simulink model "lorenz84Ver"  (R2020a)
settings: Solver=VariableStepAuto  StartTime=0.0  StopTime=25/1e5  RelTol=1e-3
undefined symbols (not defined in the file): AXI4, Lite
libraries: xbsIndex_r4 x114
settings Model: Creator=yxb20126  LastModifiedBy=yxb20126

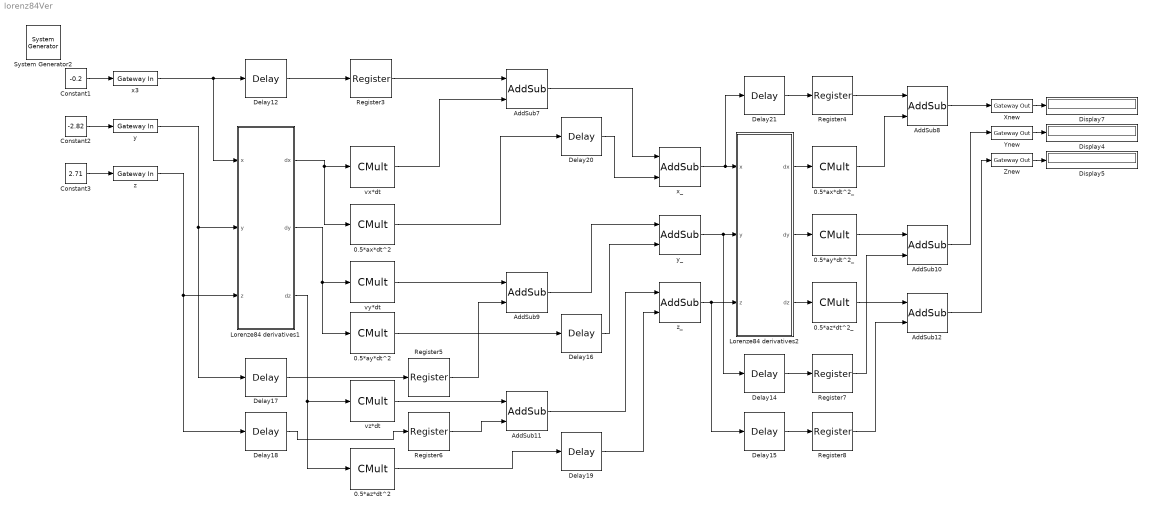
== system lorenz84Ver ==
  " System Generator2" : xbsIndex_r4/ System Generator  Tag=genX  xilinxfamily=zynq  part=xc7z020  speed=-1  package=clg400  synthesis_tool=Vivado  clock_wrapper=Clock Enables  directory=./netlist  proj_type=Vivado  Synth_file=Vivado Synthesis Defaults  Impl_file=Vivado Implementation Defaults  testbench=off  simulink_period=1/100e6  sysclk_period=10  dcm_input_clock_period=10  incr_netlist=off  trim_vbits=Everywhere in SubSystem  dbl_ovrd=According to Block Masks  core_generation=According to Block Masks  run_coregen=off  deprecated_control=off  eval_field=0  block_type=sysgen
  0.5*ax*dt^2 : xbsIndex_r4/CMult  const=5e-5  gui_display_data_type=Fixed-point  const_n_bits=32  const_bin_pt=24  float_type=Double  exp_bits=8  fraction_bits=24  en=off  latency=1  precision=User Defined  arith_type="Signed  (2's comp)"  n_bits=32  bin_pt=24  quantization=Truncate  overflow=Wrap  use_behavioral_HDL=off  mem_type=Distributed RAM  pipeline=off  dbl_ovrd=off  block_type=cmult
  0.5*ax*dt^2_ : xbsIndex_r4/CMult  const=5e-5  gui_display_data_type=Fixed-point  const_n_bits=32  const_bin_pt=24  float_type=Double  exp_bits=8  fraction_bits=24  en=off  latency=1  precision=User Defined  arith_type="Signed  (2's comp)"  n_bits=32  bin_pt=24  quantization=Truncate  overflow=Wrap  use_behavioral_HDL=off  mem_type=Distributed RAM  pipeline=off  dbl_ovrd=off  block_type=cmult
  0.5*ay*dt^2 : xbsIndex_r4/CMult  const=5e-5  gui_display_data_type=Fixed-point  const_n_bits=32  const_bin_pt=24  float_type=Double  exp_bits=8  fraction_bits=24  en=off  latency=1  precision=User Defined  arith_type="Signed  (2's comp)"  n_bits=32  bin_pt=24  quantization=Truncate  overflow=Wrap  use_behavioral_HDL=off  mem_type=Distributed RAM  pipeline=off  dbl_ovrd=off  block_type=cmult
  0.5*ay*dt^2_ : xbsIndex_r4/CMult  const=5e-5  gui_display_data_type=Fixed-point  const_n_bits=32  const_bin_pt=24  float_type=Double  exp_bits=8  fraction_bits=24  en=off  latency=1  precision=User Defined  arith_type="Signed  (2's comp)"  n_bits=32  bin_pt=24  quantization=Truncate  overflow=Wrap  use_behavioral_HDL=off  mem_type=Distributed RAM  pipeline=off  dbl_ovrd=off  block_type=cmult
  0.5*az*dt^2 : xbsIndex_r4/CMult  const=5e-5  gui_display_data_type=Fixed-point  const_n_bits=32  const_bin_pt=24  float_type=Double  exp_bits=8  fraction_bits=24  en=off  latency=1  precision=User Defined  arith_type="Signed  (2's comp)"  n_bits=32  bin_pt=24  quantization=Truncate  overflow=Wrap  use_behavioral_HDL=off  mem_type=Distributed RAM  pipeline=off  dbl_ovrd=off  block_type=cmult
  0.5*az*dt^2_ : xbsIndex_r4/CMult  const=5e-5  gui_display_data_type=Fixed-point  const_n_bits=32  const_bin_pt=24  float_type=Double  exp_bits=8  fraction_bits=24  en=off  latency=1  precision=User Defined  arith_type="Signed  (2's comp)"  n_bits=32  bin_pt=24  quantization=Truncate  overflow=Wrap  use_behavioral_HDL=off  mem_type=Distributed RAM  pipeline=off  dbl_ovrd=off  block_type=cmult
  AddSub{7..12} (6 alike) : xbsIndex_r4/AddSub  mode=Addition  use_carryin=off  use_carryout=off  en=off  latency=1  precision=User Defined  arith_type="Signed  (2's comp)"  n_bits=32  bin_pt=24  quantization=Truncate  overflow=Wrap  use_behavioral_HDL=off  hw_selection=Fabric  pipelined=off  dbl_ovrd=off  block_type=addsub
  Constant1 : Constant  Value=-0.2
  Constant2 : Constant  Value=-2.82
  Constant3 : Constant  Value=2.71
  Delay{12,14..15,17..18,21} (6 alike) : xbsIndex_r4/Delay  rst=off  infoeditControl=Selection of Reset will increase slice count due to use of real FFs and instead of SRLs  en=off  latency=15  reg_retiming=off  dbl_ovrd=off  block_type=delay
  Delay16 : xbsIndex_r4/Delay  rst=off  infoeditControl=Selection of Reset will increase slice count due to use of real FFs and instead of SRLs  en=off  latency=1  reg_retiming=off  dbl_ovrd=off  block_type=delay
  Delay19 : xbsIndex_r4/Delay  rst=off  infoeditControl=Selection of Reset will increase slice count due to use of real FFs and instead of SRLs  en=off  latency=1  reg_retiming=off  dbl_ovrd=off  block_type=delay
  Delay20 : xbsIndex_r4/Delay  rst=off  infoeditControl=Selection of Reset will increase slice count due to use of real FFs and instead of SRLs  en=off  latency=1  reg_retiming=off  dbl_ovrd=off  block_type=delay
  Display4 : Display
  Display5 : Display
  Display7 : Display
  Lorenze84 derivatives1 : Subsystem
  Lorenze84 derivatives2 : Subsystem
  Register{3..8} (6 alike) : xbsIndex_r4/Register  init=0  rst=off  en=off  dbl_ovrd=off  block_type=register
  Xnew : xbsIndex_r4/Gateway Out  inherit_from_input=off  hdl_port=on  rows=1  columns=1  UseAsDAC=off  DACChannel='1'  interface=AXI4-Lite  automatic_assignment=on  address_offset=hex2dec('00')  intf_name=''  intf_description=''  timing_constraint=None  locs_specified=off  LOCs={}  io_standard={}  block_type=gatewayout
  Ynew : xbsIndex_r4/Gateway Out  inherit_from_input=off  hdl_port=on  rows=1  columns=1  UseAsDAC=off  DACChannel='1'  interface=AXI4-Lite  automatic_assignment=on  address_offset=hex2dec('00')  intf_name=''  intf_description=''  timing_constraint=None  locs_specified=off  LOCs={}  io_standard={}  block_type=gatewayout
  Znew : xbsIndex_r4/Gateway Out  inherit_from_input=off  hdl_port=on  rows=1  columns=1  UseAsDAC=off  DACChannel='1'  interface=AXI4-Lite  automatic_assignment=on  address_offset=hex2dec('00')  intf_name=''  intf_description=''  timing_constraint=None  locs_specified=off  LOCs={}  io_standard={}  block_type=gatewayout
  vx*dt : xbsIndex_r4/CMult  const=0.01  gui_display_data_type=Fixed-point  const_n_bits=32  const_bin_pt=24  float_type=Double  exp_bits=8  fraction_bits=24  en=off  latency=1  precision=User Defined  arith_type="Signed  (2's comp)"  n_bits=32  bin_pt=24  quantization=Truncate  overflow=Wrap  use_behavioral_HDL=off  mem_type=Distributed RAM  pipeline=off  dbl_ovrd=off  block_type=cmult
  vy*dt : xbsIndex_r4/CMult  const=0.01  gui_display_data_type=Fixed-point  const_n_bits=32  const_bin_pt=24  float_type=Double  exp_bits=8  fraction_bits=24  en=off  latency=1  precision=User Defined  arith_type="Signed  (2's comp)"  n_bits=32  bin_pt=24  quantization=Truncate  overflow=Wrap  use_behavioral_HDL=off  mem_type=Distributed RAM  pipeline=off  dbl_ovrd=off  block_type=cmult
  vz*dt : xbsIndex_r4/CMult  const=0.01  gui_display_data_type=Fixed-point  const_n_bits=32  const_bin_pt=24  float_type=Double  exp_bits=8  fraction_bits=24  en=off  latency=1  precision=User Defined  arith_type="Signed  (2's comp)"  n_bits=32  bin_pt=24  quantization=Truncate  overflow=Wrap  use_behavioral_HDL=off  mem_type=Distributed RAM  pipeline=off  dbl_ovrd=off  block_type=cmult
  x3 : xbsIndex_r4/Gateway In  gui_display_data_type=Fixed-point  arith_type="Signed  (2's comp)"  n_bits=32  bin_pt=24  preci_type=Single  exp_width=8  frac_width=24  rows=1  columns=1  quantization="Round  (unbiased: +/- Inf)"  overflow=Saturate  period=1/100e6  UseAsADC=off  ADCChannel='1'  interface=AXI4-Lite  automatic_assignment=on  address_offset=hex2dec('00')  intf_name=''  intf_description=''  default_value=0  timing_constraint=None  locs_specified=off  LOCs={}  io_standard={}  inherit_from_input=off  hdl_port=on  dbl_ovrd=off  block_type=gatewayin
  x_ : xbsIndex_r4/AddSub  mode=Addition  use_carryin=off  use_carryout=off  en=off  latency=1  precision=User Defined  arith_type="Signed  (2's comp)"  n_bits=32  bin_pt=24  quantization=Truncate  overflow=Wrap  use_behavioral_HDL=off  hw_selection=Fabric  pipelined=off  dbl_ovrd=off  block_type=addsub
  y : xbsIndex_r4/Gateway In  gui_display_data_type=Fixed-point  arith_type="Signed  (2's comp)"  n_bits=32  bin_pt=24  preci_type=Single  exp_width=8  frac_width=24  rows=1  columns=1  quantization="Round  (unbiased: +/- Inf)"  overflow=Saturate  period=1/100e6  UseAsADC=off  ADCChannel='1'  interface=AXI4-Lite  automatic_assignment=on  address_offset=hex2dec('00')  intf_name=''  intf_description=''  default_value=0  timing_constraint=None  locs_specified=off  LOCs={}  io_standard={}  inherit_from_input=off  hdl_port=on  dbl_ovrd=off  block_type=gatewayin
  y_ : xbsIndex_r4/AddSub  mode=Addition  use_carryin=off  use_carryout=off  en=off  latency=1  precision=User Defined  arith_type="Signed  (2's comp)"  n_bits=32  bin_pt=24  quantization=Truncate  overflow=Wrap  use_behavioral_HDL=off  hw_selection=Fabric  pipelined=off  dbl_ovrd=off  block_type=addsub
  z : xbsIndex_r4/Gateway In  gui_display_data_type=Fixed-point  arith_type="Signed  (2's comp)"  n_bits=32  bin_pt=24  preci_type=Single  exp_width=8  frac_width=24  rows=1  columns=1  quantization="Round  (unbiased: +/- Inf)"  overflow=Saturate  period=1/100e6  UseAsADC=off  ADCChannel='1'  interface=AXI4-Lite  automatic_assignment=on  address_offset=hex2dec('00')  intf_name=''  intf_description=''  default_value=0  timing_constraint=None  locs_specified=off  LOCs={}  io_standard={}  inherit_from_input=off  hdl_port=on  dbl_ovrd=off  block_type=gatewayin
  z_ : xbsIndex_r4/AddSub  mode=Addition  use_carryin=off  use_carryout=off  en=off  latency=1  precision=User Defined  arith_type="Signed  (2's comp)"  n_bits=32  bin_pt=24  quantization=Truncate  overflow=Wrap  use_behavioral_HDL=off  hw_selection=Fabric  pipelined=off  dbl_ovrd=off  block_type=addsub
  wires:
  Constant3/1 -> z/1
  Xnew/1 -> Display7/1
  Register4/1 -> AddSub8/1
  Register5/1 -> AddSub9/2
  Delay15/1 -> Register8/1
  Lorenze84 derivatives1/2(dy) -> 0.5*ay*dt^2/1, vy*dt/1
  Lorenze84 derivatives2/2(dy) -> 0.5*ay*dt^2_/1
  x_/1 -> Lorenze84 derivatives2/1(x), Delay21/1
  x3/1 -> Lorenze84 derivatives1/1(x), Delay12/1
  Register3/1 -> AddSub7/1
  AddSub8/1 -> Xnew/1
  y_/1 -> Lorenze84 derivatives2/2(y), Delay14/1
  Register8/1 -> AddSub12/2
  Constant1/1 -> x3/1
  0.5*ay*dt^2/1 -> Delay16/1
  Delay21/1 -> Register4/1
  AddSub9/1 -> y_/1
  Delay16/1 -> y_/2
  AddSub10/1 -> Ynew/1
  Delay19/1 -> z_/2
  AddSub12/1 -> Znew/1
  0.5*ax*dt^2/1 -> Delay20/1
  Register7/1 -> AddSub10/2
  Lorenze84 derivatives1/1(dx) -> 0.5*ax*dt^2/1, vx*dt/1
  0.5*ay*dt^2_/1 -> AddSub10/1
  Delay20/1 -> x_/2
  Delay18/1 -> Register6/1
  0.5*ax*dt^2_/1 -> AddSub8/2
  AddSub11/1 -> z_/1
  z/1 -> Delay18/1, Lorenze84 derivatives1/3(z)
  vx*dt/1 -> AddSub7/2
  0.5*az*dt^2/1 -> Delay19/1
  Delay14/1 -> Register7/1
  AddSub7/1 -> x_/1
  vy*dt/1 -> AddSub9/1
  Register6/1 -> AddSub11/2
  Lorenze84 derivatives2/1(dx) -> 0.5*ax*dt^2_/1
  Delay17/1 -> Register5/1
  0.5*az*dt^2_/1 -> AddSub12/1
  vz*dt/1 -> AddSub11/1
  Znew/1 -> Display5/1
  z_/1 -> Lorenze84 derivatives2/3(z), Delay15/1
  Delay12/1 -> Register3/1
  Ynew/1 -> Display4/1
  y/1 -> Delay17/1, Lorenze84 derivatives1/2(y)
  Constant2/1 -> y/1
  Lorenze84 derivatives2/3(dz) -> 0.5*az*dt^2_/1
  Lorenze84 derivatives1/3(dz) -> 0.5*az*dt^2/1, vz*dt/1

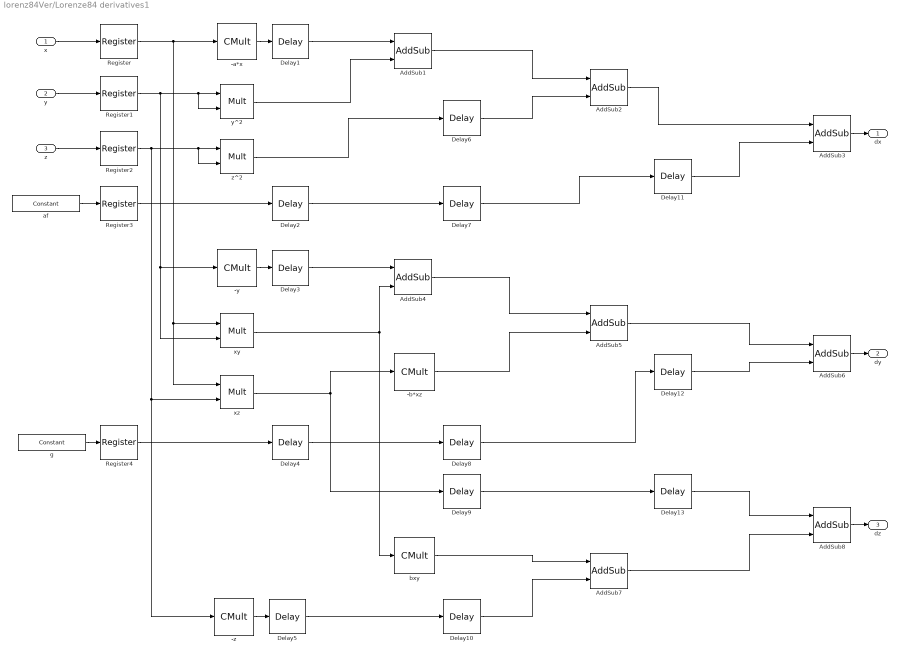
== system lorenz84Ver/Lorenze84 derivatives1 ==
  x : Inport
  y : Inport  Port=2
  z : Inport  Port=3
  -a*x : xbsIndex_r4/CMult  const=-0.95  gui_display_data_type=Fixed-point  const_n_bits=32  const_bin_pt=24  float_type=Double  exp_bits=8  fraction_bits=24  en=off  latency=1  precision=User Defined  arith_type="Signed  (2's comp)"  n_bits=32  bin_pt=24  quantization=Truncate  overflow=Wrap  use_behavioral_HDL=off  mem_type=Distributed RAM  pipeline=off  dbl_ovrd=off  block_type=cmult
  -b*xz : xbsIndex_r4/CMult  const=-7.91  gui_display_data_type=Fixed-point  const_n_bits=32  const_bin_pt=24  float_type=Double  exp_bits=8  fraction_bits=24  en=off  latency=1  precision=User Defined  arith_type="Signed  (2's comp)"  n_bits=32  bin_pt=24  quantization=Truncate  overflow=Wrap  use_behavioral_HDL=off  mem_type=Distributed RAM  pipeline=off  dbl_ovrd=off  block_type=cmult
  -y : xbsIndex_r4/CMult  const=-0.95  gui_display_data_type=Fixed-point  const_n_bits=32  const_bin_pt=24  float_type=Double  exp_bits=8  fraction_bits=24  en=off  latency=1  precision=User Defined  arith_type="Signed  (2's comp)"  n_bits=32  bin_pt=24  quantization=Truncate  overflow=Wrap  use_behavioral_HDL=off  mem_type=Distributed RAM  pipeline=off  dbl_ovrd=off  block_type=cmult
  -z : xbsIndex_r4/CMult  const=-0.95  gui_display_data_type=Fixed-point  const_n_bits=32  const_bin_pt=24  float_type=Double  exp_bits=8  fraction_bits=24  en=off  latency=1  precision=User Defined  arith_type="Signed  (2's comp)"  n_bits=32  bin_pt=24  quantization=Truncate  overflow=Wrap  use_behavioral_HDL=off  mem_type=Distributed RAM  pipeline=off  dbl_ovrd=off  block_type=cmult
  AddSub1 : xbsIndex_r4/AddSub  mode=Subtraction  use_carryin=off  use_carryout=off  en=off  latency=1  precision=User Defined  arith_type="Signed  (2's comp)"  n_bits=32  bin_pt=24  quantization=Truncate  overflow=Wrap  use_behavioral_HDL=off  hw_selection=Fabric  pipelined=off  dbl_ovrd=off  block_type=addsub
  AddSub2 : xbsIndex_r4/AddSub  mode=Subtraction  use_carryin=off  use_carryout=off  en=off  latency=1  precision=User Defined  arith_type="Signed  (2's comp)"  n_bits=32  bin_pt=24  quantization=Truncate  overflow=Wrap  use_behavioral_HDL=off  hw_selection=Fabric  pipelined=off  dbl_ovrd=off  block_type=addsub
  AddSub{3..8} (6 alike) : xbsIndex_r4/AddSub  mode=Addition  use_carryin=off  use_carryout=off  en=off  latency=1  precision=User Defined  arith_type="Signed  (2's comp)"  n_bits=32  bin_pt=24  quantization=Truncate  overflow=Wrap  use_behavioral_HDL=off  hw_selection=Fabric  pipelined=off  dbl_ovrd=off  block_type=addsub
  Delay1 : xbsIndex_r4/Delay  rst=off  infoeditControl=Selection of Reset will increase slice count due to use of real FFs and instead of SRLs  en=off  latency=2  reg_retiming=off  dbl_ovrd=off  block_type=delay
  Delay{6..13} (8 alike) : xbsIndex_r4/Delay  rst=off  infoeditControl=Selection of Reset will increase slice count due to use of real FFs and instead of SRLs  en=off  latency=1  reg_retiming=off  dbl_ovrd=off  block_type=delay
  Delay2 : xbsIndex_r4/Delay  rst=off  infoeditControl=Selection of Reset will increase slice count due to use of real FFs and instead of SRLs  en=off  latency=3  reg_retiming=off  dbl_ovrd=off  block_type=delay
  Delay3 : xbsIndex_r4/Delay  rst=off  infoeditControl=Selection of Reset will increase slice count due to use of real FFs and instead of SRLs  en=off  latency=2  reg_retiming=off  dbl_ovrd=off  block_type=delay
  Delay4 : xbsIndex_r4/Delay  rst=off  infoeditControl=Selection of Reset will increase slice count due to use of real FFs and instead of SRLs  en=off  latency=3  reg_retiming=off  dbl_ovrd=off  block_type=delay
  Delay5 : xbsIndex_r4/Delay  rst=off  infoeditControl=Selection of Reset will increase slice count due to use of real FFs and instead of SRLs  en=off  latency=2  reg_retiming=off  dbl_ovrd=off  block_type=delay
  Register{,1..4} (5 alike) : xbsIndex_r4/Register  init=0  rst=off  en=off  dbl_ovrd=off  block_type=register
  af : xbsIndex_r4/Constant  const=4.5885  gui_display_data_type=Fixed-point  arith_type=Signed (2's comp)  n_bits=32  bin_pt=24  preci_type=Double  exp_width=8  frac_width=24  explicit_period=on  period=1/100e6  equ=P=C  opselect=C  inp2=PCIN>>17  opr=+  inp1=P  carry=CIN  dbl_ovrd=off  block_type=constant
  bxy : xbsIndex_r4/CMult  const=7.91  gui_display_data_type=Fixed-point  const_n_bits=32  const_bin_pt=24  float_type=Double  exp_bits=8  fraction_bits=24  en=off  latency=1  precision=User Defined  arith_type="Signed  (2's comp)"  n_bits=32  bin_pt=24  quantization=Truncate  overflow=Wrap  use_behavioral_HDL=off  mem_type=Distributed RAM  pipeline=off  dbl_ovrd=off  block_type=cmult
  g : xbsIndex_r4/Constant  const=4.66  gui_display_data_type=Fixed-point  arith_type=Signed (2's comp)  n_bits=32  bin_pt=24  preci_type=Double  exp_width=8  frac_width=24  explicit_period=on  period=1/100e6  equ=P=C  opselect=C  inp2=PCIN>>17  opr=+  inp1=P  carry=CIN  dbl_ovrd=off  block_type=constant
  xy : xbsIndex_r4/Mult  precision=User Defined  arith_type="Signed  (2's comp)"  n_bits=32  bin_pt=24  quantization=Truncate  overflow=Wrap  en=off  latency=3  use_behavioral_HDL=off  opt=Speed  use_embedded=on  optimum_pipeline=off  pipeline=on  dbl_ovrd=off  use_rpm=on  placement_style=Triangular  block_type=mult
  xz : xbsIndex_r4/Mult  precision=User Defined  arith_type="Signed  (2's comp)"  n_bits=32  bin_pt=24  quantization=Truncate  overflow=Wrap  en=off  latency=3  use_behavioral_HDL=off  opt=Speed  use_embedded=on  optimum_pipeline=off  pipeline=on  dbl_ovrd=off  use_rpm=on  placement_style=Triangular  block_type=mult
  y^2 : xbsIndex_r4/Mult  precision=User Defined  arith_type="Signed  (2's comp)"  n_bits=32  bin_pt=24  quantization=Truncate  overflow=Wrap  en=off  latency=3  use_behavioral_HDL=off  opt=Speed  use_embedded=on  optimum_pipeline=off  pipeline=on  dbl_ovrd=off  use_rpm=on  placement_style=Triangular  block_type=mult
  z^2 : xbsIndex_r4/Mult  precision=User Defined  arith_type="Signed  (2's comp)"  n_bits=32  bin_pt=24  quantization=Truncate  overflow=Wrap  en=off  latency=3  use_behavioral_HDL=off  opt=Speed  use_embedded=on  optimum_pipeline=off  pipeline=on  dbl_ovrd=off  use_rpm=on  placement_style=Triangular  block_type=mult
  dx : Outport
  dy : Outport  Port=2
  dz : Outport  Port=3
  wires:
  y/1 -> Register1/1
  z/1 -> Register2/1
  af/1 -> Register3/1
  x/1 -> Register/1
  Register/1 -> xy/1, xz/1, -a*x/1
  Register1/1 -> xy/2, -y/1, y^2/1, y^2/2
  Register2/1 -> xz/2, -z/1, z^2/1, z^2/2
  -a*x/1 -> Delay1/1
  y^2/1 -> AddSub1/2
  AddSub1/1 -> AddSub2/1
  z^2/1 -> Delay6/1
  AddSub2/1 -> AddSub3/1
  AddSub3/1 -> dx/1
  -y/1 -> Delay3/1
  AddSub4/1 -> AddSub5/1
  -b*xz/1 -> AddSub5/2
  AddSub5/1 -> AddSub6/1
  g/1 -> Register4/1
  Register4/1 -> Delay4/1
  AddSub6/1 -> dy/1
  Register3/1 -> Delay2/1
  xy/1 -> bxy/1, AddSub4/2
  -z/1 -> Delay5/1
  bxy/1 -> AddSub7/1
  AddSub7/1 -> AddSub8/2
  xz/1 -> -b*xz/1, Delay9/1
  AddSub8/1 -> dz/1
  Delay1/1 -> AddSub1/1
  Delay2/1 -> Delay7/1
  Delay3/1 -> AddSub4/1
  Delay4/1 -> Delay8/1
  Delay5/1 -> Delay10/1
  Delay6/1 -> AddSub2/2
  Delay7/1 -> Delay11/1
  Delay8/1 -> Delay12/1
  Delay9/1 -> Delay13/1
  Delay10/1 -> AddSub7/2
  Delay11/1 -> AddSub3/2
  Delay12/1 -> AddSub6/2
  Delay13/1 -> AddSub8/1

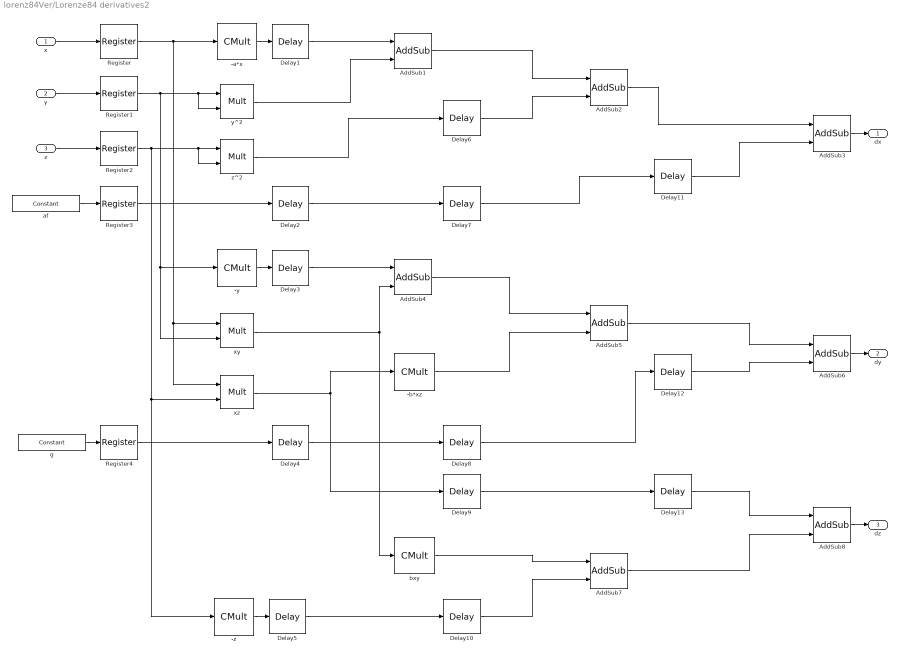
== system lorenz84Ver/Lorenze84 derivatives2 ==
  x : Inport
  y : Inport  Port=2
  z : Inport  Port=3
  -a*x : xbsIndex_r4/CMult  const=-0.95  gui_display_data_type=Fixed-point  const_n_bits=32  const_bin_pt=24  float_type=Double  exp_bits=8  fraction_bits=24  en=off  latency=1  precision=User Defined  arith_type="Signed  (2's comp)"  n_bits=32  bin_pt=24  quantization=Truncate  overflow=Wrap  use_behavioral_HDL=off  mem_type=Distributed RAM  pipeline=off  dbl_ovrd=off  block_type=cmult
  -b*xz : xbsIndex_r4/CMult  const=-7.91  gui_display_data_type=Fixed-point  const_n_bits=32  const_bin_pt=24  float_type=Double  exp_bits=8  fraction_bits=24  en=off  latency=1  precision=User Defined  arith_type="Signed  (2's comp)"  n_bits=32  bin_pt=24  quantization=Truncate  overflow=Wrap  use_behavioral_HDL=off  mem_type=Distributed RAM  pipeline=off  dbl_ovrd=off  block_type=cmult
  -y : xbsIndex_r4/CMult  const=-0.95  gui_display_data_type=Fixed-point  const_n_bits=32  const_bin_pt=24  float_type=Double  exp_bits=8  fraction_bits=24  en=off  latency=1  precision=User Defined  arith_type="Signed  (2's comp)"  n_bits=32  bin_pt=24  quantization=Truncate  overflow=Wrap  use_behavioral_HDL=off  mem_type=Distributed RAM  pipeline=off  dbl_ovrd=off  block_type=cmult
  -z : xbsIndex_r4/CMult  const=-0.95  gui_display_data_type=Fixed-point  const_n_bits=32  const_bin_pt=24  float_type=Double  exp_bits=8  fraction_bits=24  en=off  latency=1  precision=User Defined  arith_type="Signed  (2's comp)"  n_bits=32  bin_pt=24  quantization=Truncate  overflow=Wrap  use_behavioral_HDL=off  mem_type=Distributed RAM  pipeline=off  dbl_ovrd=off  block_type=cmult
  AddSub1 : xbsIndex_r4/AddSub  mode=Subtraction  use_carryin=off  use_carryout=off  en=off  latency=1  precision=User Defined  arith_type="Signed  (2's comp)"  n_bits=32  bin_pt=24  quantization=Truncate  overflow=Wrap  use_behavioral_HDL=off  hw_selection=Fabric  pipelined=off  dbl_ovrd=off  block_type=addsub
  AddSub2 : xbsIndex_r4/AddSub  mode=Subtraction  use_carryin=off  use_carryout=off  en=off  latency=1  precision=User Defined  arith_type="Signed  (2's comp)"  n_bits=32  bin_pt=24  quantization=Truncate  overflow=Wrap  use_behavioral_HDL=off  hw_selection=Fabric  pipelined=off  dbl_ovrd=off  block_type=addsub
  AddSub{3..8} (6 alike) : xbsIndex_r4/AddSub  mode=Addition  use_carryin=off  use_carryout=off  en=off  latency=1  precision=User Defined  arith_type="Signed  (2's comp)"  n_bits=32  bin_pt=24  quantization=Truncate  overflow=Wrap  use_behavioral_HDL=off  hw_selection=Fabric  pipelined=off  dbl_ovrd=off  block_type=addsub
  Delay1 : xbsIndex_r4/Delay  rst=off  infoeditControl=Selection of Reset will increase slice count due to use of real FFs and instead of SRLs  en=off  latency=2  reg_retiming=off  dbl_ovrd=off  block_type=delay
  Delay{6..13} (8 alike) : xbsIndex_r4/Delay  rst=off  infoeditControl=Selection of Reset will increase slice count due to use of real FFs and instead of SRLs  en=off  latency=1  reg_retiming=off  dbl_ovrd=off  block_type=delay
  Delay2 : xbsIndex_r4/Delay  rst=off  infoeditControl=Selection of Reset will increase slice count due to use of real FFs and instead of SRLs  en=off  latency=3  reg_retiming=off  dbl_ovrd=off  block_type=delay
  Delay3 : xbsIndex_r4/Delay  rst=off  infoeditControl=Selection of Reset will increase slice count due to use of real FFs and instead of SRLs  en=off  latency=2  reg_retiming=off  dbl_ovrd=off  block_type=delay
  Delay4 : xbsIndex_r4/Delay  rst=off  infoeditControl=Selection of Reset will increase slice count due to use of real FFs and instead of SRLs  en=off  latency=3  reg_retiming=off  dbl_ovrd=off  block_type=delay
  Delay5 : xbsIndex_r4/Delay  rst=off  infoeditControl=Selection of Reset will increase slice count due to use of real FFs and instead of SRLs  en=off  latency=2  reg_retiming=off  dbl_ovrd=off  block_type=delay
  Register{,1..4} (5 alike) : xbsIndex_r4/Register  init=0  rst=off  en=off  dbl_ovrd=off  block_type=register
  af : xbsIndex_r4/Constant  const=4.5885  gui_display_data_type=Fixed-point  arith_type=Signed (2's comp)  n_bits=32  bin_pt=24  preci_type=Double  exp_width=8  frac_width=24  explicit_period=on  period=1/100e6  equ=P=C  opselect=C  inp2=PCIN>>17  opr=+  inp1=P  carry=CIN  dbl_ovrd=off  block_type=constant
  bxy : xbsIndex_r4/CMult  const=7.91  gui_display_data_type=Fixed-point  const_n_bits=32  const_bin_pt=24  float_type=Double  exp_bits=8  fraction_bits=24  en=off  latency=1  precision=User Defined  arith_type="Signed  (2's comp)"  n_bits=32  bin_pt=24  quantization=Truncate  overflow=Wrap  use_behavioral_HDL=off  mem_type=Distributed RAM  pipeline=off  dbl_ovrd=off  block_type=cmult
  g : xbsIndex_r4/Constant  const=4.66  gui_display_data_type=Fixed-point  arith_type=Signed (2's comp)  n_bits=32  bin_pt=24  preci_type=Double  exp_width=8  frac_width=24  explicit_period=on  period=1/100e6  equ=P=C  opselect=C  inp2=PCIN>>17  opr=+  inp1=P  carry=CIN  dbl_ovrd=off  block_type=constant
  xy : xbsIndex_r4/Mult  precision=User Defined  arith_type="Signed  (2's comp)"  n_bits=32  bin_pt=24  quantization=Truncate  overflow=Wrap  en=off  latency=3  use_behavioral_HDL=off  opt=Speed  use_embedded=on  optimum_pipeline=off  pipeline=on  dbl_ovrd=off  use_rpm=on  placement_style=Triangular  block_type=mult
  xz : xbsIndex_r4/Mult  precision=User Defined  arith_type="Signed  (2's comp)"  n_bits=32  bin_pt=24  quantization=Truncate  overflow=Wrap  en=off  latency=3  use_behavioral_HDL=off  opt=Speed  use_embedded=on  optimum_pipeline=off  pipeline=on  dbl_ovrd=off  use_rpm=on  placement_style=Triangular  block_type=mult
  y^2 : xbsIndex_r4/Mult  precision=User Defined  arith_type="Signed  (2's comp)"  n_bits=32  bin_pt=24  quantization=Truncate  overflow=Wrap  en=off  latency=3  use_behavioral_HDL=off  opt=Speed  use_embedded=on  optimum_pipeline=off  pipeline=on  dbl_ovrd=off  use_rpm=on  placement_style=Triangular  block_type=mult
  z^2 : xbsIndex_r4/Mult  precision=User Defined  arith_type="Signed  (2's comp)"  n_bits=32  bin_pt=24  quantization=Truncate  overflow=Wrap  en=off  latency=3  use_behavioral_HDL=off  opt=Speed  use_embedded=on  optimum_pipeline=off  pipeline=on  dbl_ovrd=off  use_rpm=on  placement_style=Triangular  block_type=mult
  dx : Outport
  dy : Outport  Port=2
  dz : Outport  Port=3
  wires:
  Delay13/1 -> AddSub8/1
  Delay12/1 -> AddSub6/2
  Delay11/1 -> AddSub3/2
  Delay10/1 -> AddSub7/2
  Delay9/1 -> Delay13/1
  Delay8/1 -> Delay12/1
  Delay7/1 -> Delay11/1
  Delay6/1 -> AddSub2/2
  Delay5/1 -> Delay10/1
  Delay4/1 -> Delay8/1
  Delay3/1 -> AddSub4/1
  Delay2/1 -> Delay7/1
  Delay1/1 -> AddSub1/1
  AddSub8/1 -> dz/1
  xz/1 -> Delay9/1, -b*xz/1
  AddSub7/1 -> AddSub8/2
  bxy/1 -> AddSub7/1
  -z/1 -> Delay5/1
  xy/1 -> AddSub4/2, bxy/1
  Register3/1 -> Delay2/1
  AddSub6/1 -> dy/1
  Register4/1 -> Delay4/1
  g/1 -> Register4/1
  AddSub5/1 -> AddSub6/1
  -b*xz/1 -> AddSub5/2
  AddSub4/1 -> AddSub5/1
  -y/1 -> Delay3/1
  AddSub3/1 -> dx/1
  AddSub2/1 -> AddSub3/1
  z^2/1 -> Delay6/1
  AddSub1/1 -> AddSub2/1
  y^2/1 -> AddSub1/2
  -a*x/1 -> Delay1/1
  Register2/1 -> z^2/2, z^2/1, -z/1, xz/2
  Register1/1 -> y^2/2, y^2/1, -y/1, xy/2
  Register/1 -> -a*x/1, xz/1, xy/1
  x/1 -> Register/1
  af/1 -> Register3/1
  z/1 -> Register2/1
  y/1 -> Register1/1
